simulink model "Model_40_01_2"  (R2024b)
settings: Solver=VariableStepAuto  StartTime=0.0  StopTime=50  RelTol=1e-3
undefined symbols (not defined in the file): kd, ki, kp, z03
libraries: slpidlib x1
settings Model: Creator=ricki  LastModifiedBy=ricki

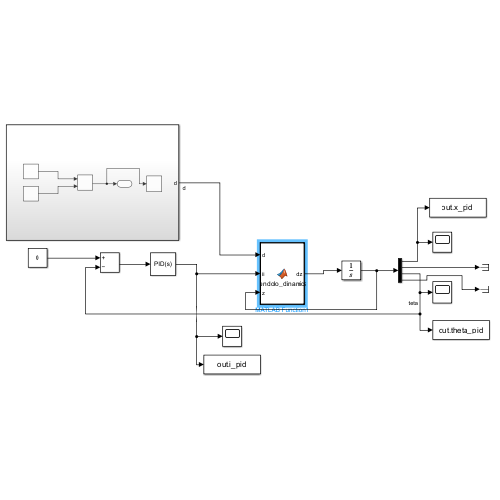
[thumbnail: Simulink's stored preview of the top-level diagram]
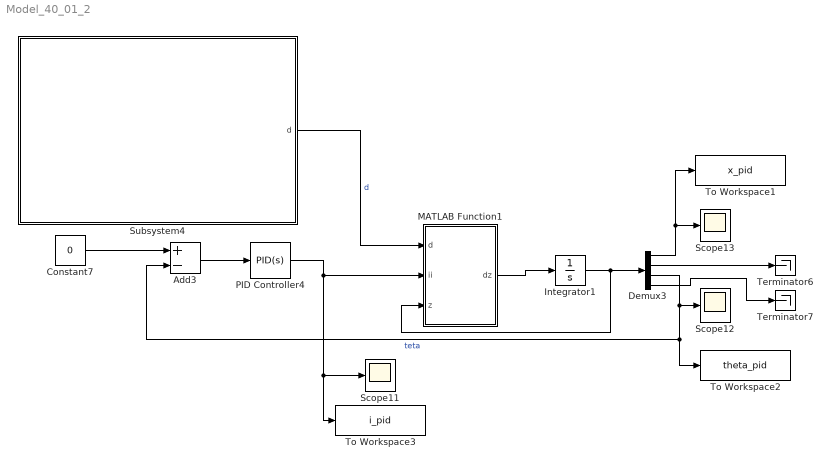
== system Model_40_01_2 ==
  Add3 : Sum  Inputs=+-
  Constant7 : Constant  Value=0
  Demux3 : Demux
  Integrator1 : Integrator  InitialCondition=z03  AbsoluteTolerance=1e-4
  MATLAB Function1 : MATLAB Function  TreatAsAtomicUnit=on
  PID Controller4 : slpidlib/PID Controller  Controller=PID  Form=Parallel  TimeDomain=Continuous-time  UseExternalTs=off  SampleTime=-1  IntegratorMethod=Forward Euler  FilterMethod=Forward Euler  ControllerParametersSource=internal  P=kp  I=ki  UseKiTs=off  D=kd  UseExternalDerivativeSource=off  N=100  UseFilter=on  TunerSelectOption=Transfer Function Based (PID Tuner App)  InitialConditionSource=internal  InitialConditionForIntegrator=0  InitialConditionForFilter=0  DifferentiatorICPrevScaledInput=0  ExternalReset=none  TrackingMode=off  Kt=1  LimitOutput=off  SatLimitsSource=internal  UpperSaturationLimit=inf  LowerSaturationLimit=-inf  LinearizeAsGain=on  AntiWindupMode=none  Kb=1  LimitIntegrator=off  UpperIntegratorSaturationLimit=inf  LowerIntegratorSaturationLimit=-inf  POutMin=[]  POutMax=[]  IOutMin=[]  IOutMax=[]  DOutMin=[]  DOutMax=[]  NOutMin=[]  NOutMax=[]  SumOutMin=[]  SumOutMax=[]  SaturationOutMin=[]  SaturationOutMax=[]  PParamMin=[]  PParamMax=[]  IParamMin=[]  IParamMax=[]  DParamMin=[]  DParamMax=[]  NParamMin=[]  NParamMax=[]  KbParamMin=[]  KbParamMax=[]  KtParamMin=[]  KtParamMax=[]  KbOutMin=[]  KbOutMax=[]  KtOutMin=[]  KtOutMax=[]  IntegratorOutMin=[]  IntegratorOutMax=[]  FilterOutMin=[]  FilterOutMax=[]  SumI1OutMin=[]  SumI1OutMax=[]  SumI2OutMin=[]  SumI2OutMax=[]  SumI3OutMin=[]  SumI3OutMax=[]  SumI4OutMin=[]  SumI4OutMax=[]  SumDOutMin=[]  SumDOutMax=[]  DifferentiatorOutMin=[]  DifferentiatorOutMax=[]  FilterDiffOutCoefMin=[]  FilterDiffOutCoefMax=[]  ReciprocalOutMin=[]  ReciprocalOutMax=[]  SumDenOutMin=[]  SumDenOutMax=[]  SumNumOutMin=[]  SumNumOutMax=[]  DivideOutMin=[]  DivideOutMax=[]  UdiffTsProdOutMin=[]  UdiffTsProdOutMax=[]  NTsProdOutMin=[]  NTsProdOutMax=[]  UintegralTsProdOutMin=[]  UintegralTsProdOutMax=[]  UngainTsProdOutMin=[]  UngainTsProdOutMax=[]  ClampingZeroOutDataTypeStr=Inherit: Inherit via back propagation  ClampingZeroOutMin=[]  ClampingZeroOutMax=[]  FilterDenConstantOutDataTypeStr=Inherit: Inherit via back propagation  FilterDenConstantOutMin=[]  FilterDenConstantOutMax=[]  PCopyOutDataTypeStr=Inherit: Inherit via back propagation  PCopyOutMin=[]  PCopyOutMax=[]  NCopyOutDataTypeStr=Inherit: Inherit via back propagation  NCopyOutMin=[]  NCopyOutMax=[]  IntegratorContinuousStateAttributes=''  IntegratorStateMustResolveToSignalObject=off  IntegratorRTWStateStorageClass=Auto  FilterContinuousStateAttributes=''  FilterStateMustResolveToSignalObject=off  FilterRTWStateStorageClass=Auto  ParallelPVariant=InternalParameters  IdealPVariant=Disabled  IVariant=InternalParameters  DVariant=InternalParameters  IntegratorVariant=Continuous  SatVariant=Disabled  AWVariant=Passthrough  PCopyVariant=Disabled  TRVariant=Disabled  FdbkBlocksVariant=Forward  IdealPFdbkVariant=Disabled  SatFdbkVariant=Disabled  DerivativeFilterVariant=ContFilter  NVariant=InternalParameters  NCopyVariant=Disabled  FilterICVariant=InternalICsFilter  IntegratorICVariant=InternalICs  ExternalResetVariant=Disabled  TRSumVariant=Passthrough  SumFdbkVariant=Disabled  SumVariant=Sum_PID  TsampFilterVariant=InternalTs  TsampNgainVariant=Passthrough  TsampIntegralVariant=Disabled_SignalSpec  ExternalSaturationOutDataTypeStr=Inherit: Same as second input  DerivativeSourceVariant=ErrorSignal  PreIntVariant=InternalPreInt
  Scope11 : Scope
  Scope12 : Scope
  Scope13 : Scope
  Subsystem4 : Subsystem
  Terminator6 : Terminator
  Terminator7 : Terminator
  To Workspace1 : ToWorkspace  VariableName=x_pid  SampleTime=-1
  To Workspace2 : ToWorkspace  VariableName=theta_pid  SampleTime=-1
  To Workspace3 : ToWorkspace  VariableName=i_pid  SampleTime=-1
  wires:
  Demux3/4 -> Terminator7/1
  Subsystem4/1(d) -> MATLAB Function1/1(d)  "d"
  Demux3/2 -> Terminator6/1
  Integrator1/1 -> MATLAB Function1/3(z), Demux3/1
  Demux3/1 -> To Workspace1/1, Scope13/1
  PID Controller4/1 -> To Workspace3/1, Scope11/1, MATLAB Function1/2(ii)
  Constant7/1 -> Add3/1
  MATLAB Function1/1(dz) -> Integrator1/1
  Add3/1 -> PID Controller4/1
  Demux3/3 -> To Workspace2/1, Add3/2, Scope12/1  "teta"

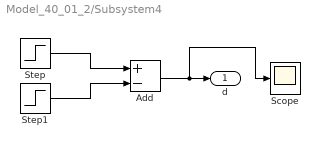
== system Model_40_01_2/Subsystem4 ==
  Add : Sum  Inputs=+-
  Scope : Scope
  Step : Step  SampleTime=0
  Step1 : Step  Time=3  SampleTime=0
  d : Outport
  wires:
  Step/1 -> Add/1
  Step1/1 -> Add/2
  Add/1 -> Scope/1, d/1

== matlab function Model_40_01_2/MATLAB Function1 ==
  data: d input; ii input; dz output; z input; lab1P parameter
function dz = pendolo_dinamica(d, ii, z, lab1P)
% 
% Calcola la derivata del vettore di stato valutando il sistema controllato 
% tramite una legge di retroazione di stato parziale
% considerando la presenza di attriti.


%definisco un denominatore comune
den=(lab1P.I0*lab1P.I2 - lab1P.I1^2*cos(z(3))^2 + lab1P.I2*lab1P.M);
%sistema del punto 1.3
dz=[z(2);
    -(- lab1P.g*sin(z(3))*lab1P.I1^2*cos(z(3)) + lab1P.I2*sin(z(3))*lab1P.I1*z(4)^2 + lab1P.b*lab1P.I1*z(4)*cos(z(3)) - lab1P.alpha1*d*lab1P.I1*cos(z(3))^2 + lab1P.I2*lab1P.alpha0*d - lab1P.I2*lab1P.alpham*ii + lab1P.I2*lab1P.c*z(2))/den;
    z(4);
    -(lab1P.I0*lab1P.b*z(4) + lab1P.M*lab1P.b*z(4) - lab1P.I0*lab1P.I1*lab1P.g*sin(z(3)) - lab1P.I1*lab1P.M*lab1P.g*sin(z(3)) - lab1P.I0*lab1P.alpha1*d*cos(z(3)) + lab1P.I1*lab1P.alpha0*d*cos(z(3)) - lab1P.M*lab1P.alpha1*d*cos(z(3)) - lab1P.I1*lab1P.alpham*ii*cos(z(3)) + lab1P.I1*lab1P.c*z(2)*cos(z(3)) + lab1P.I1^2*z(4)^2*cos(z(3))*sin(z(3)))/den];

end
